simulink model "ctrlauto_tp1_f"  (R2019b)
settings: Solver=ode45  StartTime=0.0  StopTime=1  FixedStep=0.001  RelTol=1e-3
undefined symbols (not defined in the file or in its folder): K, ueq, x0, xeq, yref
settings Model: Creator=aghersin  LastModifiedBy=rochi
settings DataIOCC: ReturnWorkspaceOutputs=off
settings DebuggingCC: ArithmeticOperatorsInVariantConditions=warning
settings SFSimCC: SimUseLocalCustomCode=off  CustomCodeUndefinedFunction=UseInterfaceOnly
settings RTWCC: RTWUseLocalCustomCode=off

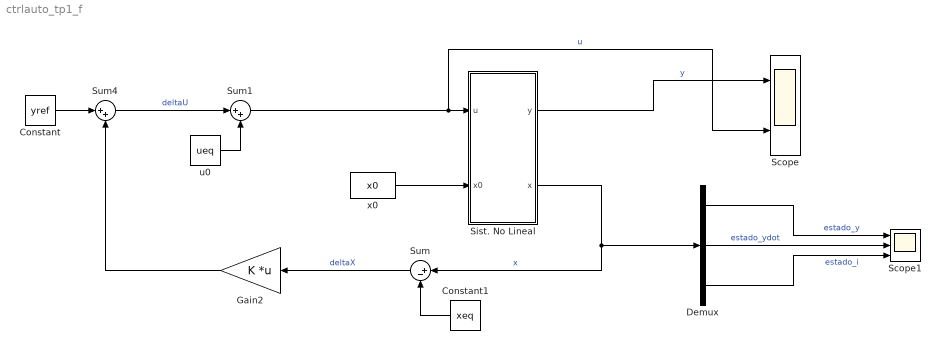
== system ctrlauto_tp1_f ==
  Constant : Constant  Value=yref
  Constant1 : Constant  Value=xeq
  Demux : Demux  Outputs=3
  Gain2 : Gain  Gain=K  Multiplication=Matrix(K*u)
  Scope : Scope  NumInputPorts=2
  Scope1 : Scope  NumInputPorts=3
  "Sist. No Lineal " : Subsystem
  Sum : Sum  Inputs=|+-
  Sum1 : Sum  Inputs=|++
  Sum4 : Sum  Inputs=|++
  u0 : Constant  Value=ueq
  x0 : Constant  Value=x0
  wires:
  Gain2/1 -> Sum4/2
  Sum4/1 -> Sum1/1  "deltaU"
  u0/1 -> Sum1/2
  Sum1/1 -> Scope/2, "Sist. No Lineal "/1(u)  "u"
  Constant/1 -> Sum4/1
  "Sist. No Lineal "/1(y) -> Scope/1  "y"
  x0/1 -> "Sist. No Lineal "/2(x0)
  Sum/1 -> Gain2/1  "deltaX"
  Constant1/1 -> Sum/2
  "Sist. No Lineal "/2(x) -> Sum/1, Demux/1  "x"
  Demux/3 -> Scope1/3  "estado_i"
  Demux/1 -> Scope1/1  "estado_y"
  Demux/2 -> Scope1/2  "estado_ydot"

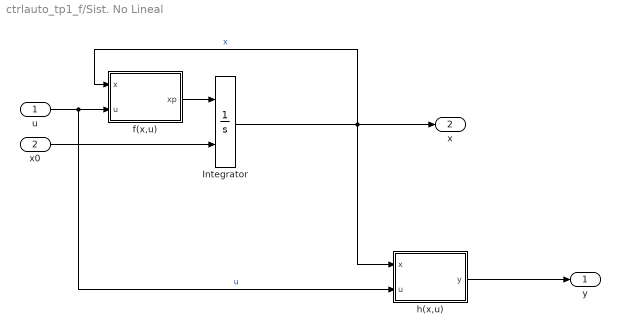
== system ctrlauto_tp1_f/Sist. No Lineal  ==
  u : Inport
  x0 : Inport  Port=2
  Integrator : Integrator  InitialConditionSource=external  ZeroCross=off
  f(x,u) : MATLAB Function  TreatAsAtomicUnit=on
  h(x,u) : MATLAB Function  TreatAsAtomicUnit=on
  y : Outport  VectorParamsAs1DForOutWhenUnconnected=off
  x : Outport  Port=2  VectorParamsAs1DForOutWhenUnconnected=off
  wires:
  h(x,u)/1(y) -> y/1
  u/1 -> h(x,u)/2(u), f(x,u)/2(u)  "u"
  f(x,u)/1(xp) -> Integrator/1
  Integrator/1 -> h(x,u)/1(x), x/1, f(x,u)/1(x)  "x"
  x0/1 -> Integrator/2

== matlab function ctrlauto_tp1_f/Sist. No Lineal /f(x,u) ==
  data: x input; u input; xp output
function xp = f(x,u)

xp1 = x(2);
xp2 = (5*(x(3) + 2)^2)/(2*(x(1) - 1)^2) ...
    - (5*(x(3) - 2)^2)/(2*(x(1) + 1)^2) - 10; 
xp3 = - 4*x(3)^2 + u;

xp = [xp1; xp2; xp3];

== matlab function ctrlauto_tp1_f/Sist. No Lineal /h(x,u) ==
  data: x input; u input; y output
function y = h(x,u)

y=x(1);
